simulink model "Dashboard"  (R2019a)
settings: Solver=VariableStepAuto  StartTime=0.0  StopTime=inf  RelTol=1e-3
settings Model: Creator=anton  LastModifiedBy=anton

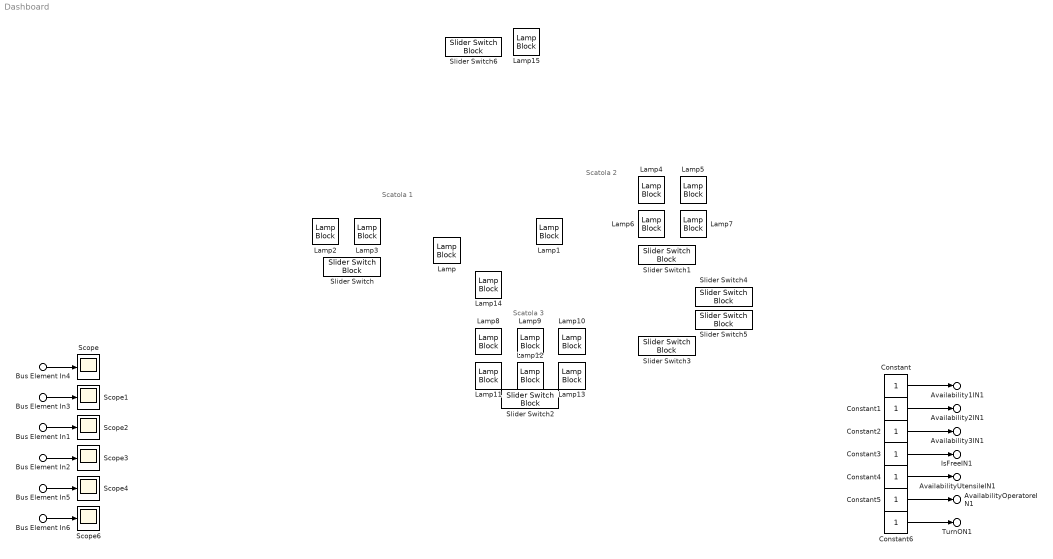
== system Dashboard ==
  note: Scatola 1
  note: Scatola 2
  note: Scatola 3
  Bus Element In1 : Inport  PortName=Capienza1IN
  Bus Element In2 : Inport  Port=2  PortName=Capienza2IN
  Bus Element In3 : Inport  Port=3  PortName=Capienza3IN
  Bus Element In4 : Inport  Port=4  PortName=Pick1Completed
  Bus Element In5 : Inport  Port=5  PortName=Pick2Completed
  Bus Element In6 : Inport  Port=6  PortName=Pick3Completed
  Constant{,1..6} (7 alike) : Constant
  Lamp{,1..15} (16 alike) : LampBlock
  Scope{,1..4,6} (6 alike) : Scope
  Slider Switch{,1..6} (7 alike) : SliderSwitchBlock
      settings: Values={{'Off', 'On'}, [0 1]}
  TurnON1 : Outport  PortName=TurnON
  AvailabilityOperatoreIN1 : Outport  Port=2  PortName=AvailabilityOperatoreIN
  Availability1IN1 : Outport  Port=3  PortName=Availability1IN
  Availability2IN1 : Outport  Port=4  PortName=Availability2IN
  AvailabilityUtensileIN1 : Outport  Port=5  PortName=AvailabilityUtensileIN
  IsFreeIN1 : Outport  Port=6  PortName=IsFreeIN
  Availability3IN1 : Outport  Port=7  PortName=Availability3IN
  wires:
  Constant1/1 -> Availability2IN1/1
  Constant4/1 -> AvailabilityUtensileIN1/1
  Constant3/1 -> IsFreeIN1/1
  Bus Element In4/1 -> Scope/1
  Constant5/1 -> AvailabilityOperatoreIN1/1
  Constant/1 -> Availability1IN1/1
  Bus Element In1/1 -> Scope2/1
  Bus Element In2/1 -> Scope3/1
  Bus Element In6/1 -> Scope6/1
  Constant2/1 -> Availability3IN1/1
  Constant6/1 -> TurnON1/1
  Bus Element In3/1 -> Scope1/1
  Bus Element In5/1 -> Scope4/1
